simulink model "phase1_PRControl_CIM_Adapt"  (R2024a)
settings: Solver=VariableStepAuto  StartTime=0.0  StopTime=20  FixedStep=1e-6  MaxStep=1e-6  RelTol=1e-6
values from neighbouring files (symbols this model uses):
  alpha_adapt = 100    [phase1_PRControl_CIM_Adapt_init.m]
  Am0_can = sys0_ocf.A    [phase1_PRControl_CIM_Adapt_init.m]
  Bm1_can = sys1_ocf.B    [phase1_PRControl_CIM_Adapt_init.m]
  c_adapt = 0.1    [phase1_PRControl_CIM_Adapt_init.m]
  Cf = 22e-6    (= 2.2e-05)    [phase1_PRControl_CIM_Adapt_init.m]
  Cm0_can = sys0_ocf.C    [phase1_PRControl_CIM_Adapt_init.m]
  E = 1    [phase1_PRControl_CIM_Adapt_init.m]
  freq = 49.5    [phase1_PRControl_CIM_Adapt_init.m]
  L1 = 150e-6    (= 0.00015)    [phase1_PRControl_CIM_Adapt_init.m]
  L2g = L2+Lg    (= 0.00045)    [phase1_PRControl_CIM_Adapt_init.m]
  m_m1 = size(Bm1_can,2)    [phase1_PRControl_CIM_Adapt_init.m]
  n_m0 = size(Am0_can,1)    [phase1_PRControl_CIM_Adapt_init.m]
  p_e = size(E,1)    [phase1_PRControl_CIM_Adapt_init.m]
  PiInit = k0_adapt*eye(m_m1)    [phase1_PRControl_CIM_Adapt_init.m]
  Q_adapt = zeros(m_m1,1)    [phase1_PRControl_CIM_Adapt_init.m]
  R1 = 0.045    [phase1_PRControl_CIM_Adapt_init.m]
  R2g = R2+Rg    (= 0.135)    [phase1_PRControl_CIM_Adapt_init.m]
  Rd = 1    [phase1_PRControl_CIM_Adapt_init.m]
  Theta0 = w0^2    (= 98696.0440109)    [phase1_PRControl_CIM_Adapt_init.m]
  w = 2*pi*freq    (= 311.017672705)    [phase1_PRControl_CIM_Adapt_init.m]
undefined symbols (not defined in the file or in its folder): alfa, Am0, beta, Bm1, C_filter, Cm1, DiscIntNeverNeededParam, Dm1, Down, dt, n0, nu, Th_bar, Up
libraries: fl_lib x34, nesl_utility x23, ee_lib x9, spsSeriesRLCBranchLib x9, cstblocks x7, spsVoltageMeasurementLib x5, spsCurrentMeasurementLib x2, spsDCVoltageSourceLib x2, simulink x2, spsACVoltageSourceLib x1, spsControlledVoltageSourceLib x1, spsBreakerLib x1
(part 1 of 2)
settings Model: Creator=aleks  LastModifiedBy=aleks
settings DataIOCC: ReturnWorkspaceOutputs=off
settings SimscapeCC: SimscapeLogType=all  SimscapeLogOpenViewer=on  SimscapeLogLimitData=off

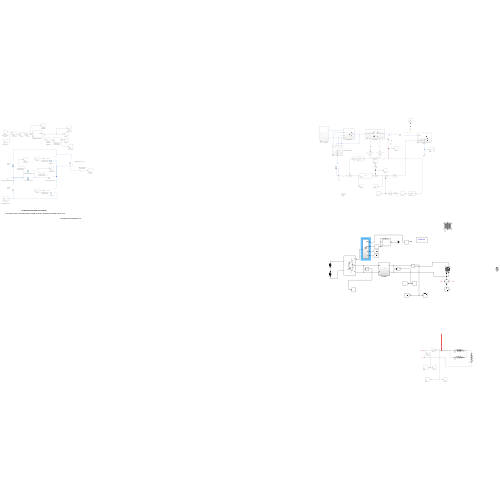
[thumbnail: Simulink's stored preview of the top-level diagram]
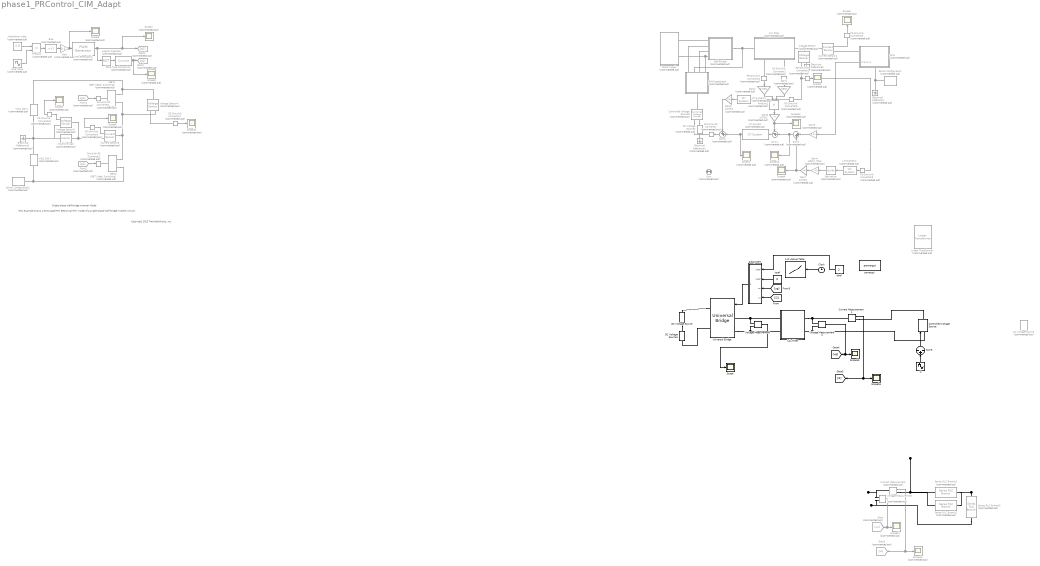
== system phase1_PRControl_CIM_Adapt ==
  note: Single-phase Half-bridge Inverter Model
  note: Copyright 2023 The MathWorks, Inc.
  note: This example shows a Simscape(TM) Electrical(TM) model of a single-phase half-bridge inverter circuit.
  1-D Lookup Table : Lookup_n-D  NumberOfTableDimensions=1  LookupTableObject=''  BreakpointsForDimension1=[0;0.2;0.201;3]  BreakpointsForDimension1FirstPoint=10  BreakpointsForDimension2FirstPoint=10  BreakpointsForDimension1Spacing=12  BreakpointsForDimension2Spacing=12  IndexSearchMethod=Linear search  Table=[0;0;2;2]  DiagnosticForOutOfRangeInput=Error  InternalRulePriority=Speed  RndMeth=Simplest
  AC Voltage Source : spsACVoltageSourceLib/AC Voltage Source  Commented=on  Amplitude=15  Phase=0  Frequency=freq  SampleTime=0  Measurements=None  BusType=swing  Pref=10e3  Qref=0  Qmin=-inf  Qmax=+inf
  Bias : Bias  Commented=on  Bias=1  SaturateOnIntegerOverflow=off
  Clock : Clock
  Controlled Voltage Source2 : fl_lib/Electrical/Electrical Sources/Controlled Voltage Source  Commented=on
  Controlled Voltage Source : spsControlledVoltageSourceLib/Controlled Voltage Source  Initialize=on  Source_Type=AC  Amplitude=0  Phase=0  Frequency=0  Measurements=None
  Current Measurement : spsCurrentMeasurementLib/Current Measurement  Commented=on  PhasorSimulation=off  OutputType=Complex  PSBequivalent=0
  Current Measurement1 : spsCurrentMeasurementLib/Current Measurement  PhasorSimulation=off  OutputType=Complex  PSBequivalent=0
  Current Sensor3 : fl_lib/Electrical/Electrical Sensors/Current Sensor  Commented=on
  Current Sensor4 : fl_lib/Electrical/Electrical Sensors/Current Sensor  Commented=on
  DC Voltage Source : spsDCVoltageSourceLib/DC Voltage Source  Amplitude=20  Measurements=None
  DC Voltage Source1 : spsDCVoltageSourceLib/DC Voltage Source  Amplitude=20  Measurements=None
  DC Voltage Source2 : ee_lib/Additional Components/SPICE Sources/DC Voltage Source  Commented=on  DC=0.3 V
  Data Type Conversion : DataTypeConversion  Commented=on  SaturateOnIntegerOverflow=off  RndMeth=Floor
  Derivative : Derivative  Commented=on
  Electrical Reference{,1..3} (4 alike) : fl_lib/Electrical/Electrical Elements/Electrical Reference  Commented=on
  From1 : From  Commented=on  GotoTag=g1
  From2 : From  Commented=on  GotoTag=g2
  Gain : Gain  Commented=on  Gain=0.5
  Gain1 : Gain  Commented=on  Gain=beta
  Gain2 : Gain  Commented=on  Gain=1-beta
  Gain3 : Gain  Commented=on  Gain=0.01
  Gain4 : Gain  Commented=on  Gain=alfa*C_filter
  Gain5 : Gain  Commented=on  Gain=1/370/2
  Gain6 : Gain  Commented=on  Gain=1/370/2
  Gain7 : Gain  Commented=on  Gain=1/370/2
  Goto : Goto  Commented=on  GotoTag=uo
  Goto1 : Goto  Commented=on  GotoTag=g1
  Goto2 : Goto  Commented=on  GotoTag=g2
  Goto3 : Goto  Commented=on  GotoTag=io
  Grid : Subsystem  Commented=on
      settings: PortSchema="{\"entries\":[{\"content\":{\"sides\":[{\"content\":{\"connectorIds\":[\"LConn1\",\"Out1\"]},\"type\":\"ConnectorPlacement.EquallySpacedRectSide\",\"uuid\":\"60da00de-121a-44fc-8184-3f94833a613b\"},{\"content\":{\"side\":\"RIGHT\"},\"type\":\"ConnectorPlacement.EquallySpacedRectSide\",\"uuid\":\"59ba5a48-7211-453f-9bde-add9e34e0a3d\"},{\"content\":{\"side\":\"TOP\"},\"type\":\"ConnectorPlacement.EquallySpacedRectSide\",\"uuid\":\"7a4f9c1b-94f2-4e83-81a9-ee65f7316222\"},{\"content\":{\"connectorIds\":[\"RConn1\"],\"side\":\"BOTTOM\"},\"type\":\"ConnectorPlacement.EquallySpacedRectSide\",\"uuid\":\"6582cb16-51de-4783-ba21-138861469b9e\"}]},\"type\":\"ConnectorPlacement.EquallySpacedConnector\",\"uuid\":\"6f9c893a-ff6e-44db-92a9-569068b12591\"}],\"packageUris\":[\"http://schema.mathworks.com/mf0/Connector/R2020b\"],\"version\":\"1.0\"}"
  Half-Bridge : Subsystem  Commented=on
  IGBT1 : ee_lib/Semiconductors & Converters/IGBT (Ideal, Switching)  Commented=on  port_option=ee.enum.controlport.ps  Vf=0.8 V  Ron=0.001 Ohm  Goff=1e-5 1/Ohm  Vth=0.5 V  diode_param=2  diode_Vf=0.8 V  diode_Ron=0.001 Ohm  diode_Goff=1e-5 1/Ohm  diode_C=50e-9 F  diode_iRM=-235 A  diode_iF=300 A  diode_idot=-50 A/us  diode_trr_param=1  diode_trr_factor=3  diode_trr=15 us  diode_Qrr=1500 s*uA  ice_specify=off  ice_priority=None  ice=0 A  ice_nominal_specify=off  ice_nominal_value=1  ice_nominal_unit=A  vce_specify=off  vce_priority=None  vce=0 V  vce_nominal_specify=off  vce_nominal_value=1  vce_nominal_unit=V  vge_specify=off  vge_priority=None  vge=0 V  vge_nominal_specify=off  vge_nominal_value=1  vge_nominal_unit=V  thermal_loss_option=ee.enum.converters.thermalLossOption.constantvalues  Von_data=[0, .1, .6, .8, 1, 1.3, 1.6, 2, 2.4; 0, .1, .7, 1, 1.2, 1.5, 1.9, 2.4, 2.8] V  Tj=[298.15, 398.15] K  Iout_data=[0, .1, 1, 5, 10, 20, 40, 70, 100] A  Eon_data=[0, .0024, .024, .12, .2, .48, 1.04, 2.16, 3.24; 0, .003, .03, .15, .25, .6, 1.3, 2.7, 4.05] * 1e-3 J  Eoff_data=[0, .0007, .0066, .033, .066, .17, .33, .83, 1.5; 0, .001, .01, .05, .1, .25, .5, 1.2, 2.2] * 1e-3 J  Eon_data_3D=[zeros(2, 9, 3)] J  Eoff_data_3D=[zeros(2, 9, 3)] J  Tj_loss=[298.15, 398.15] K  Iout_data_loss=[0, .1, 1, 5, 10, 20, 40, 70, 100] A  tabulateWithVce=false  Vce_loss=[0, 150, 300] V  Eon_scalar=22.86e-3 J  Eoff_scalar=17.14e-3 J  Voff=300 V  Iout_scalar=600 A  useCurrentFromPreviousCycle=false  useVoltageFromPreviousCycle=false  diodeModelType=ee.enum.converters.diodeModelType.pwl  diodeTableType=ee.enum.diode.tableType.IfMat  diode_ReverseIVType=ee.enum.diode.diodeReverseIV.constant  diode_IfMat=[.07, .12, .19, 1.75, 4.24, 7.32, 11.2; .16, .3, .72, 2.14, 4.02, 6.35, 9.12] A  diode_VfMat=[.9, 1.15, 1.25, 1.5, 1.75, 2.17, 2.6, 2.85; .58, .68, .75, 1.1, 1.38, 1.77, 2.27, 2.7] V  diode_TjVec=[25, 125] degC  diode_VfVec=[.5, .7, .9, 1.3, 1.7, 2.1, 2.5] V  diode_IfVec=[.1, .2, .5, 1, 2, 4, 7, 10] A  diode_IrMat=[1e-06, 2e-06, 5e-06, 1e-05, 2.5e-05, 5e-05, .0001; 2e-06, 5e-06, 1e-05, 4e-05, 8e-05, .0002, .0005] A  diode_VrMat=[10, 100, 200, 250, 300, 325, 350; 10, 70, 160, 220, 270, 300, 320] V  diode_VrVec=[10, 20, 40, 50, 70, 80, 100] V  diode_IrVec=[1e-06, 2e-06, 5e-06, 1e-05, 2e-05, 5e-05, .0001] A  diode_Vr=-600 V  diode_Ls=150 nH  diode_Erec=0.03 J  diode_rec_loss_model=ee.enum.diode.reverseRecoveryModel.fixed  diode_ErecVal=0 J  diode_scaleWithIandV=true  diode_ErecMat=zeros(2, 3) J  diode_TjrecVec=[298.15, 398.15] K  diode_IfrecVec=[.1, 1, 10] A  diode_IrecVal=10 A  diode_VrecVal=10 V  diode_tFilter=1 / 1000 / 100 s  thermal_network_parameterization=ee.enum.thermalNetworkTopology.external  Rth=[.08, .5] K/W  Rth_Cauer=[.08, .1, .5] K/W  Rth_Foster=[.08, .14, .22, .16] K/W  thermal_mass_parameterization=ee.enum.thermalNetwork.timeconstant  thermal_mass=[.01, .5] J/K  thermal_mass_Cauer=[.01, .1, .5] J/K  thermal_mass_Foster=[.001, .005, .05, .5] J/K  thermal_time_constant=[.001, .2] s  thermal_time_constant_Cauer=[.001, .1, .2] s  thermal_time_constant_Foster=[7e-05, .0007, .01, .08] s  thermal_mass_initial_temperatures=[25, 25] degC  thermal_mass_initial_temperatures_Cauer=[25, 25, 25] degC  junction_thermal_mass=0.01 J/K  Tvec_initial_Foster=[25, 25, 25, 25] degC  no_thermal_network=0  junction_temperature_specify=off  junction_temperature_priority=None  junction_temperature=25 degC  junction_temperature_nominal_specify=off  junction_temperature_nominal_value=1  junction_temperature_nominal_unit=degC  Qj_specify=off  Qj_priority=None  Qj=0 W  Qj_nominal_specify=off  Qj_nominal_value=1  Qj_nominal_unit=W  accumulatedSwitchingLosses_specify=off  accumulatedSwitchingLosses_priority=None  accumulatedSwitchingLosses=0 J
  IGBT2 : ee_lib/Semiconductors & Converters/IGBT (Ideal, Switching)  Commented=on  port_option=ee.enum.controlport.ps  Vf=0.8 V  Ron=0.001 Ohm  Goff=1e-5 1/Ohm  Vth=0.5 V  diode_param=2  diode_Vf=0.8 V  diode_Ron=0.001 Ohm  diode_Goff=1e-5 1/Ohm  diode_C=50e-9 F  diode_iRM=-235 A  diode_iF=300 A  diode_idot=-50 A/us  diode_trr_param=1  diode_trr_factor=3  diode_trr=15 us  diode_Qrr=1500 s*uA  ice_specify=off  ice_priority=None  ice=0 A  ice_nominal_specify=off  ice_nominal_value=1  ice_nominal_unit=A  vce_specify=off  vce_priority=None  vce=0 V  vce_nominal_specify=off  vce_nominal_value=1  vce_nominal_unit=V  vge_specify=off  vge_priority=None  vge=0 V  vge_nominal_specify=off  vge_nominal_value=1  vge_nominal_unit=V  thermal_loss_option=ee.enum.converters.thermalLossOption.constantvalues  Von_data=[0, .1, .6, .8, 1, 1.3, 1.6, 2, 2.4; 0, .1, .7, 1, 1.2, 1.5, 1.9, 2.4, 2.8] V  Tj=[298.15, 398.15] K  Iout_data=[0, .1, 1, 5, 10, 20, 40, 70, 100] A  Eon_data=[0, .0024, .024, .12, .2, .48, 1.04, 2.16, 3.24; 0, .003, .03, .15, .25, .6, 1.3, 2.7, 4.05] * 1e-3 J  Eoff_data=[0, .0007, .0066, .033, .066, .17, .33, .83, 1.5; 0, .001, .01, .05, .1, .25, .5, 1.2, 2.2] * 1e-3 J  Eon_data_3D=[zeros(2, 9, 3)] J  Eoff_data_3D=[zeros(2, 9, 3)] J  Tj_loss=[298.15, 398.15] K  Iout_data_loss=[0, .1, 1, 5, 10, 20, 40, 70, 100] A  tabulateWithVce=false  Vce_loss=[0, 150, 300] V  Eon_scalar=22.86e-3 J  Eoff_scalar=17.14e-3 J  Voff=300 V  Iout_scalar=600 A  useCurrentFromPreviousCycle=false  useVoltageFromPreviousCycle=false  diodeModelType=ee.enum.converters.diodeModelType.pwl  diodeTableType=ee.enum.diode.tableType.IfMat  diode_ReverseIVType=ee.enum.diode.diodeReverseIV.constant  diode_IfMat=[.07, .12, .19, 1.75, 4.24, 7.32, 11.2; .16, .3, .72, 2.14, 4.02, 6.35, 9.12] A  diode_VfMat=[.9, 1.15, 1.25, 1.5, 1.75, 2.17, 2.6, 2.85; .58, .68, .75, 1.1, 1.38, 1.77, 2.27, 2.7] V  diode_TjVec=[25, 125] degC  diode_VfVec=[.5, .7, .9, 1.3, 1.7, 2.1, 2.5] V  diode_IfVec=[.1, .2, .5, 1, 2, 4, 7, 10] A  diode_IrMat=[1e-06, 2e-06, 5e-06, 1e-05, 2.5e-05, 5e-05, .0001; 2e-06, 5e-06, 1e-05, 4e-05, 8e-05, .0002, .0005] A  diode_VrMat=[10, 100, 200, 250, 300, 325, 350; 10, 70, 160, 220, 270, 300, 320] V  diode_VrVec=[10, 20, 40, 50, 70, 80, 100] V  diode_IrVec=[1e-06, 2e-06, 5e-06, 1e-05, 2e-05, 5e-05, .0001] A  diode_Vr=-600 V  diode_Ls=150 nH  diode_Erec=0.03 J  diode_rec_loss_model=ee.enum.diode.reverseRecoveryModel.fixed  diode_ErecVal=0 J  diode_scaleWithIandV=true  diode_ErecMat=zeros(2, 3) J  diode_TjrecVec=[298.15, 398.15] K  diode_IfrecVec=[.1, 1, 10] A  diode_IrecVal=10 A  diode_VrecVal=10 V  diode_tFilter=1 / 1000 / 100 s  thermal_network_parameterization=ee.enum.thermalNetworkTopology.external  Rth=[.08, .5] K/W  Rth_Cauer=[.08, .1, .5] K/W  Rth_Foster=[.08, .14, .22, .16] K/W  thermal_mass_parameterization=ee.enum.thermalNetwork.timeconstant  thermal_mass=[.01, .5] J/K  thermal_mass_Cauer=[.01, .1, .5] J/K  thermal_mass_Foster=[.001, .005, .05, .5] J/K  thermal_time_constant=[.001, .2] s  thermal_time_constant_Cauer=[.001, .1, .2] s  thermal_time_constant_Foster=[7e-05, .0007, .01, .08] s  thermal_mass_initial_temperatures=[25, 25] degC  thermal_mass_initial_temperatures_Cauer=[25, 25, 25] degC  junction_thermal_mass=0.01 J/K  Tvec_initial_Foster=[25, 25, 25, 25] degC  no_thermal_network=0  junction_temperature_specify=off  junction_temperature_priority=None  junction_temperature=25 degC  junction_temperature_nominal_specify=off  junction_temperature_nominal_value=1  junction_temperature_nominal_unit=degC  Qj_specify=off  Qj_priority=None  Qj=0 W  Qj_nominal_specify=off  Qj_nominal_value=1  Qj_nominal_unit=W  accumulatedSwitchingLosses_specify=off  accumulatedSwitchingLosses_priority=None  accumulatedSwitchingLosses=0 J
  Idref : Constant  Value=2
  Inductive load : fl_lib/Electrical/Electrical Elements/Inductor  Commented=on  l=0.005 H  r=1 Ohm  g=0 1/Ohm  i_specify=off  i_priority=None  i=0 A  i_nominal_specify=off  i_nominal_value=1  i_nominal_unit=A  v_specify=off  v_priority=None  v=0 V  v_nominal_specify=off  v_nominal_value=1  v_nominal_unit=V  i_L_specify=off  i_L_priority=High  i_L=0 A  i_L_nominal_specify=off  i_L_nominal_value=1  i_L_nominal_unit=A
  Iqref : Constant  Value=0
  LCL Filter : Subsystem
  LCL filter : Subsystem  Commented=on
      settings: PortSchema="{\"entries\":[{\"content\":{\"sides\":[{\"content\":{\"connectorIds\":[\"LConn1\"]},\"type\":\"ConnectorPlacement.EquallySpacedRectSide\",\"uuid\":\"8b3831d8-2af2-4e09-98b8-6e5c23c190ef\"},{\"content\":{\"connectorIds\":[\"RConn1\"],\"side\":\"RIGHT\"},\"type\":\"ConnectorPlacement.EquallySpacedRectSide\",\"uuid\":\"7bed20d9-2cda-4fdb-ba4d-dd3d87999dd3\"},{\"content\":{\"side\":\"TOP\"},\"type\":\"ConnectorPlacement.EquallySpacedRectSide\",\"uuid\":\"ddfcc6a1-9f78-4bcc-aaa8-1a77e264e72f\"},{\"content\":{\"connectorIds\":[\"RConn2\",\"RConn3\"],\"side\":\"BOTTOM\"},\"type\":\"ConnectorPlacement.EquallySpacedRectSide\",\"uuid\":\"a456a5b4-e9ed-42f1-ab5a-c7df7a648cd2\"}]},\"type\":\"ConnectorPlacement.EquallySpacedConnector\",\"uuid\":\"6c992da4-40d5-4809-a728-0540f255a39b\"}],\"packageUris\":[\"http://schema.mathworks.com/mf0/Connector/R2020b\"],\"version\":\"1.0\"}"
  LTI System : cstblocks/LTI System  Commented=on  sys=Gpr  IC=[]  PadeOrder=0
  LTI System1 : cstblocks/LTI System  Commented=on  sys=Gfffilter  IC=[]  PadeOrder=0
  LTI System2 : cstblocks/LTI System  Commented=on  sys=Gfffilter  IC=[]  PadeOrder=0
  Linear Transformer : spsLinearTransformerLib/Linear Transformer  Commented=on  UNITS=pu  NominalPower=[ 45 50 ]  winding1="[ 15/sqrt(2)  0.002  0.01 ]"  winding2="[ 230  0.002  0.01 ]"  ThreeWindings=off  winding3=[ 315e3 0.002 0.08 ]  RmLm=[ 500 500 ]  Measurements=None  DataType=off
  Logical Operator : Logic  Commented=on  Operator=NOT  AllPortsSameDT=off  OutDataTypeStr=boolean
  Modulation Index : Constant  Commented=on  Value=0.8
  PS-Simulink Converter{1..9} (9 alike) : nesl_utility/PS-Simulink Converter  Commented=on  PhysicalDomain=network_engine_domain  SubClassName=ps_output  LeftPortType=input  RightPortType=output  PseudoPeriodic=off  Frequencies=[]  VectorFormat=inherit  Unit=inherit  AffineConversion=off
  PWM Generator1 : eePwmGenerator/PWM Generator  Commented=on  CarrCount=Up-Down  Tper=1/2/2000  Tdelay=0  Ts=0
  PWM generator : Subsystem  Commented=on
  Power supply : Subsystem  Commented=on
  Product : Product  Commented=on  RndMeth=Zero
  Product1 : Product  Commented=on
  Scope : Scope
  Scope{1..14} (14 alike) : Scope  Commented=on
  Scope15 : Scope
  Scope16 : Scope
  Series RLC Branch1 : spsSeriesRLCBranchLib/Series RLC Branch  Commented=on  LConnTagsString=__new0  RConnTagsString=__new0  BranchType=L  Resistance=0.053  Inductance=5e-3  SetiL0=off  InitialCurrent=0  Capacitance=1e-6  Setx0=off  InitialVoltage=0  Measurements=None
  Series RLC Branch2 : spsSeriesRLCBranchLib/Series RLC Branch  Commented=on  LConnTagsString=__new0  RConnTagsString=__new0  BranchType=R  Resistance=500  Inductance=500e-6  SetiL0=off  InitialCurrent=0  Capacitance=1e-6  Setx0=off  InitialVoltage=0  Measurements=None
  Series RLC Branch3 : spsSeriesRLCBranchLib/Series RLC Branch  Commented=on  LConnTagsString=__new0  RConnTagsString=__new0  BranchType=R  Resistance=5  Inductance=500e-6  SetiL0=off  InitialCurrent=0  Capacitance=1e-6  Setx0=off  InitialVoltage=0  Measurements=None
  Simulink-PS Converter : nesl_utility/Simulink-PS Converter  Commented=on  PhysicalDomain=network_engine_domain  SubClassName=ps_input  LeftPortType=input  RightPortType=output  PseudoPeriodic=off  Frequencies=[]  NoiseDistribution=none  NoiseParameters=[]  Unit=1  AffineConversion=off  FilteringAndDerivatives=provide  SimscapeFilterOrder=1  InputFilterTimeConstant=0.001  UdotUserProvided=0
  Simulink-PS Converter1 : nesl_utility/Simulink-PS Converter  Commented=on  PhysicalDomain=network_engine_domain  SubClassName=ps_input  LeftPortType=input  RightPortType=output  PseudoPeriodic=off  Frequencies=[]  NoiseDistribution=none  NoiseParameters=[]  Unit=1  AffineConversion=off  FilteringAndDerivatives=provide  SimscapeFilterOrder=1  InputFilterTimeConstant=0.001  UdotUserProvided=0
  Simulink-PS Converter2 : nesl_utility/Simulink-PS Converter  Commented=on  PhysicalDomain=network_engine_domain  SubClassName=ps_input  LeftPortType=input  RightPortType=output  PseudoPeriodic=off  Frequencies=[]  NoiseDistribution=none  NoiseParameters=[]  Unit=1  AffineConversion=off  FilteringAndDerivatives=provide  SimscapeFilterOrder=1  InputFilterTimeConstant=0.001  UdotUserProvided=0
  Sine Wave : Sin  Commented=on  Frequency=2*pi*50  SampleTime=0
  Solver Configuration : nesl_utility/Solver Configuration  Commented=on  PhysicalDomain=network_engine_domain  SubClassName=solver  LeftPortType=input  RightPortType=generic  Tones=[]  Harmonics=[]  SimulateNoise=off  Profile=off  UseLocalSampling=off  EnableSwitchedLinearOptims=on  FrequencyDomain=off  UseCCode=off  RelTol=0.001  AbsTol=0.001  MinStep=1e-09  ToWorkspace=off  RevertToSquareIcSolve=off  NumHomotopyIterations=100  PhasorMode=off  PhasorModeNumHarmonics=1  ConsistencySolver=NEWTON_XTOL_AFTER_FTOL  IndexReductionMethod=DerivativeReplacement  DoDC=off  ResidualTolerance=1e-09  ConsistencyTolSource=GLOBAL  ConsistencyAbsTol=0.001  ConsistencyRelTol=0.001  ConsistencyTolFactor=0.001  UseLocalSolver=off  LocalSolverChoice=NE_BACKWARD_EULER_ADVANCER  ResolveIndetEquations=on  FunctionEvalNumThread=1  LocalSolverSampleTime=0.001  DoFixedCost=off  MaxNonlinIter=3  MaxModeIter=2  ComputeImpulses=off  ImpulseIterations=2  LinearAlgebra=auto  LinearAlgebraNumThread=0  EquationFormulation=NE_TIME_EF  DelaysMemoryBudget=1024  AutomaticFiltering=on  FilteringTimeConstant=0.001  PartitionStorageMethod=AS_NEEDED  PartitionMemoryBudget=1024  PartitionMethod=ROBUST  MultibodyUseLocalSolver=off  MultibodyLocalSolverChoice=ODE1  MultibodyLocalSolverSampleTime=0.001
  Solver Configuration2 : nesl_utility/Solver Configuration  Commented=on  PhysicalDomain=network_engine_domain  SubClassName=solver  LeftPortType=input  RightPortType=generic  Tones=[]  Harmonics=[]  SimulateNoise=off  Profile=off  UseLocalSampling=off  EnableSwitchedLinearOptims=on  FrequencyDomain=off  UseCCode=off  RelTol=0.001  AbsTol=1e-06  MinStep=1e-09  ToWorkspace=off  RevertToSquareIcSolve=off  NumHomotopyIterations=100  PhasorMode=off  PhasorModeNumHarmonics=1  ConsistencySolver=NEWTON_FTOL  IndexReductionMethod=DerivativeReplacement  DoDC=off  ResidualTolerance=1e-09  ConsistencyTolSource=GLOBAL  ConsistencyAbsTol=0.001  ConsistencyRelTol=0.001  ConsistencyTolFactor=0.001  UseLocalSolver=off  LocalSolverChoice=NE_BACKWARD_EULER_ADVANCER  ResolveIndetEquations=on  FunctionEvalNumThread=1  LocalSolverSampleTime=5e-05  DoFixedCost=off  MaxNonlinIter=3  MaxModeIter=2  ComputeImpulses=off  ImpulseIterations=1  LinearAlgebra=Sparse  LinearAlgebraNumThread=0  EquationFormulation=NE_TIME_EF  DelaysMemoryBudget=1024  AutomaticFiltering=on  FilteringTimeConstant=0.001  PartitionStorageMethod=AS_NEEDED  PartitionMemoryBudget=1024  PartitionMethod=FAST  MultibodyUseLocalSolver=off  MultibodyLocalSolverChoice=ODE1  MultibodyLocalSolverSampleTime=0.001
  Subsystem : Subsystem
  Sum : Sum  Commented=on  Inputs=+|+
  Sum1 : Sum  Commented=on  Inputs=-+|
  Sum2 : Sum  Commented=on  Inputs=|++
  Sum3 : Sum  Commented=on  Inputs=++|
  Sum5 : Sum  Inputs=-|+|-
  Universal Bridge : spsUniversalBridgeLib/Universal Bridge  Arms=2  SnubberResistance=1e5  SnubberCapacitance=inf  Device=IGBT / Diodes  Ron=1e-3  Lon=0  ForwardVoltages="[  0  0  ]"  ForwardVoltage=0  GTOparameters=[ 10e-6 , 20e-6 ]  IGBTparameters=[ 1e-6 , 2e-6 ]  Measurements=None  Measurements_2=None  converterType=Rectifier
  Vdc1 100 V : fl_lib/Electrical/Electrical Sources/DC Voltage Source  Commented=on  v0=100 V
  Vdc2 100 V : fl_lib/Electrical/Electrical Sources/DC Voltage Source  Commented=on  v0=100 V
  Voltage Measurement : spsVoltageMeasurementLib/Voltage Measurement  PhasorSimulation=off  OutputType=Complex  PSBequivalent=0
  Voltage Measurement1 : spsVoltageMeasurementLib/Voltage Measurement  Commented=on  PhasorSimulation=off  OutputType=Complex  PSBequivalent=0
  Voltage Measurement2 : spsVoltageMeasurementLib/Voltage Measurement  PhasorSimulation=off  OutputType=Complex  PSBequivalent=0
  Voltage Sensor : fl_lib/Electrical/Electrical Sensors/Voltage Sensor  Commented=on
  Voltage Sensor3 : fl_lib/Electrical/Electrical Sensors/Voltage Sensor  Commented=on
  Voltage Sensor4 : fl_lib/Electrical/Electrical Sensors/Voltage Sensor  Commented=on
  powergui : spspowerguiLib/powergui  Priority=1  SimulationMode=Continuous  SampleTime=10e-6  frequency=60  Iterations=50  frequencyindice=0  Pbase=100e6  ErrMax=1e-4  UnitsV=kV  UnitsW=MW  buscounter=0  FunctionMessages=off  echomessages=off  EnableUseOfTLC=off  CurrentSourceSwitches=off  DisableSnubberDevices=off  DisableRonSwitches=off  DisableVfSwitches=off  DisplayEquations=off  AutomaticDiscreteSolvers=off  SolverType=Tustin/Backward Euler (TBE)  Interpol=off  ExternalGateDelay=off  methode=off  Ts=100  x0status=blocks  SPID=on  SwTol=0  HookPort=off  NonlinearTolerance=1e-4  nMaxIteration=100  ContinueOnMaxIteration=off  RestoreLinks=warning  ResistiveCurrentMeasurement=off  Frange=[0:2:500]  Ylog=off  Xlog=on  ShowGrid=off  save=off  variable=ZData  structure=0  ZoomFFT=off  StartTime=0.0  cycles=1  DisplayStyle=1  fundamental=60  FreqAxis=off  MaxFrequency=1000  frequencyindicesteady=1  RmsSteady=1  display=off
  w : Sin  Amplitude=15  Frequency=w  SampleTime=0
  wires:
  PS-Simulink Converter2/1 -> Scope2/1
  Bias/1 -> Gain/1
  Product/1 -> Bias/1
  From1/1 -> Simulink-PS Converter1/1
  Logical Operator/1 -> Data Type Conversion/1
  Sine Wave/1 -> Product/2
  PS-Simulink Converter5/1 -> Scope6/1
  From2/1 -> Simulink-PS Converter2/1
  PS-Simulink Converter6/1 -> Scope5/1
  Modulation Index/1 -> Product/1
  Data Type Conversion/1 -> Scope9/1, Goto2/1
  PWM Generator1/1 -> Scope7/1, Goto1/1, Logical Operator/1
  Gain/1 -> Scope8/1, PWM Generator1/1
  PS-Simulink Converter7/1 -> Scope10/1
  PS-Simulink Converter3/1 -> Scope3/1
  PS-Simulink Converter1/1 -> Gain1/1
  PS-Simulink Converter4/1 -> Gain2/1
  Gain2/1 -> Product1/1
  Gain1/1 -> Product1/2
  Grid/1(sinewave) -> Gain3/1
  Gain3/1 -> Sum2/1
  Gain6/1 -> Sum1/1, Scope13/1
  Sum1/1 -> LTI System/1
  Derivative/1 -> Gain4/1
  Gain7/1 -> Sum2/2, Scope4/1
  Sum2/1 -> Scope12/1, Sum1/2
  LTI System/1 -> Sum3/2, Scope1/1
  PS-Simulink Converter8/1 -> LTI System1/1
  Sum3/1 -> Simulink-PS Converter/1
  Gain5/1 -> Sum3/1
  Product1/1 -> Gain6/1
  LTI System1/1 -> Gain5/1
  PS-Simulink Converter9/1 -> LTI System2/1
  LTI System2/1 -> Derivative/1
  Gain4/1 -> Gain7/1
  Voltage Measurement/1 -> Scope/1
  Subsystem/1(1) -> Universal Bridge/1
  [i2] -> Subsystem/4(io)
  [ug] -> Subsystem/3(uo)
  Current Measurement/1 -> Scope14/1, Goto3/1
  Voltage Measurement1/1 -> Goto/1, Scope11/1
  Voltage Measurement2/1 -> [ug], Scope15/1
  Current Measurement1/1 -> Scope16/1, [i2]
  w/1 -> Sum5/2
  ? -> ?
  ? -> ?
  Sum5/1 -> Controlled Voltage Source/1
  Iqref/1 -> Subsystem/2(iqref)
  Idref/1 -> Subsystem/1(idref)
  Clock/1 -> 1-D Lookup Table/1
  connections:
  Voltage Sensor/LConn1 -- Current Sensor4/LConn1 -- LCL filter/RConn1
  Voltage Sensor/RConn1 -- PS-Simulink Converter9/LConn1 -- PS-Simulink Converter8/LConn1 -- PS-Simulink Converter2/LConn1
  Solver Configuration2/RConn1 -- Vdc2 100 V/RConn1 -- IGBT2/RConn2
  Vdc1 100 V/RConn1 -- Vdc2 100 V/LConn1 -- Electrical Reference2/LConn1 -- Inductive load/RConn1 -- Voltage Sensor3/RConn2
  Current Sensor3/RConn2 -- Inductive load/LConn1 -- Voltage Sensor3/LConn1
  IGBT2/RConn1 -- Current Sensor3/LConn1 -- IGBT1/RConn2 -- Voltage Sensor4/RConn2
  IGBT1/RConn1 -- Voltage Sensor4/LConn1 -- Vdc1 100 V/LConn1
  PS-Simulink Converter5/LConn1 -- Current Sensor3/RConn1
  PS-Simulink Converter6/LConn1 -- Voltage Sensor3/RConn1
  IGBT2/LConn1 -- Simulink-PS Converter2/RConn1
  IGBT1/LConn1 -- Simulink-PS Converter1/RConn1
  Voltage Sensor4/RConn1 -- PS-Simulink Converter7/LConn1
  Controlled Voltage Source2/LConn1 -- PWM generator/LConn1
  Half-Bridge/RConn1 -- PWM generator/RConn2 -- LCL filter/LConn1
  Half-Bridge/LConn2 -- PWM generator/RConn1
  PWM generator/RConn3 -- Half-Bridge/LConn3
  Voltage Sensor/RConn2 -- Electrical Reference3/LConn1
  PS-Simulink Converter3/LConn1 -- Current Sensor4/RConn1
  Current Sensor4/RConn2 -- Grid/LConn1
  Electrical Reference/LConn1 -- Solver Configuration/RConn1 -- Grid/RConn1
  PWM generator/RConn4 -- Power supply/RConn2 -- Half-Bridge/LConn4
  Half-Bridge/LConn1 -- Power supply/RConn1
  DC Voltage Source2/RConn1 -- Electrical Reference1/LConn1
  Controlled Voltage Source2/RConn2 -- DC Voltage Source2/LConn1
  PS-Simulink Converter4/LConn1 -- LCL filter/RConn2
  LCL filter/RConn3 -- PS-Simulink Converter1/LConn1
  Controlled Voltage Source2/RConn1 -- Simulink-PS Converter/RConn1
  Universal Bridge/RConn1 -- DC Voltage Source/RConn1
  Universal Bridge/RConn2 -- DC Voltage Source1/LConn1
  Voltage Measurement/LConn1 -- LCL Filter/LConn1 -- Universal Bridge/LConn1
  Voltage Measurement2/LConn2 -- Controlled Voltage Source/LConn1 -- LCL Filter/RConn2
  DC Voltage Source/LConn1 -- DC Voltage Source1/RConn1
  Voltage Measurement1/LConn1 -- Current Measurement/LConn1
  Series RLC Branch1/LConn1 -- Series RLC Branch2/LConn1 -- Current Measurement/RConn1
  Series RLC Branch3/LConn1 -- Series RLC Branch1/RConn1 -- Series RLC Branch2/RConn1
  Series RLC Branch3/RConn1 -- Voltage Measurement1/LConn2
  Voltage Measurement2/LConn1 -- LCL Filter/RConn1 -- Current Measurement1/LConn1
  Voltage Measurement/LConn2 -- LCL Filter/LConn2 -- Universal Bridge/LConn2
  Current Measurement1/RConn1 -- Controlled Voltage Source/RConn1

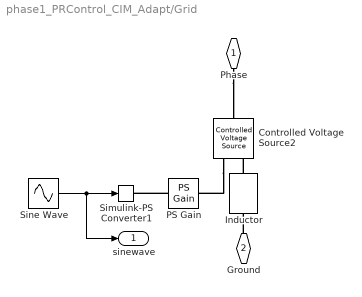
== system phase1_PRControl_CIM_Adapt/Grid ==
  Controlled Voltage Source2 : fl_lib/Electrical/Electrical Sources/Controlled Voltage Source
  Inductor : fl_lib/Electrical/Electrical Elements/Inductor  l=5e-3 H  r=0.35 Ohm  g=1e-9 1/Ohm  i_specify=off  i_priority=None  i=0 A  i_nominal_specify=off  i_nominal_value=1  i_nominal_unit=A  v_specify=off  v_priority=None  v=0 V  v_nominal_specify=off  v_nominal_value=1  v_nominal_unit=V  i_L_specify=off  i_L_priority=High  i_L=0 A  i_L_nominal_specify=off  i_L_nominal_value=1  i_L_nominal_unit=A
  PS Gain : fl_lib/Physical Signals/Functions/PS Gain  gain=220
  Simulink-PS Converter1 : nesl_utility/Simulink-PS Converter  PhysicalDomain=network_engine_domain  SubClassName=ps_input  LeftPortType=input  RightPortType=output  PseudoPeriodic=off  Frequencies=[]  NoiseDistribution=none  NoiseParameters=[]  Unit=1  AffineConversion=off  FilteringAndDerivatives=filter  SimscapeFilterOrder=1  InputFilterTimeConstant=0.0001  UdotUserProvided=0
  Sine Wave : Sin  Frequency=2*pi*50  SampleTime=0
  Phase : PMIOPort  Side=Left
  Ground : PMIOPort  Port=2  Side=Right
  sinewave : Outport
  wires:
  Sine Wave/1 -> sinewave/1, Simulink-PS Converter1/1
  connections:
  Phase/RConn1 -- Controlled Voltage Source2/LConn1
  Controlled Voltage Source2/RConn1 -- PS Gain/RConn1
  Inductor/LConn1 -- Controlled Voltage Source2/RConn2
  Ground/RConn1 -- Inductor/RConn1
  PS Gain/LConn1 -- Simulink-PS Converter1/RConn1

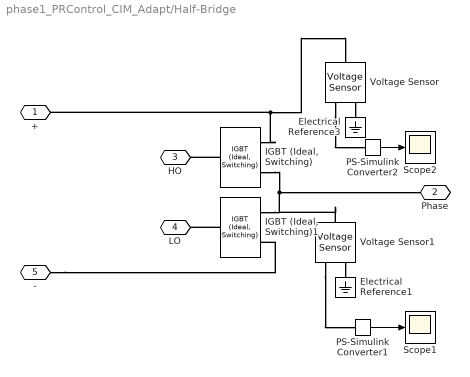
== system phase1_PRControl_CIM_Adapt/Half-Bridge ==
  Electrical Reference1 : fl_lib/Electrical/Electrical Elements/Electrical Reference
  Electrical Reference3 : fl_lib/Electrical/Electrical Elements/Electrical Reference
  "IGBT (Ideal, Switching)" : ee_lib/Semiconductors & Converters/IGBT (Ideal, Switching)  port_option=ee.enum.controlport.elec  Vf=0.8 V  Ron=0.001 Ohm  Goff=1e-5 1/Ohm  Vth=0.5 V  diode_param=ee.enum.semiconductors.protectionDiode.nodynamics  diode_Vf=0.8 V  diode_Ron=0.001 Ohm  diode_Goff=1e-5 1/Ohm  diode_C=50e-9 F  diode_iRM=-235 A  diode_iF=300 A  diode_idot=-50 A/us  diode_trr_param=ee.enum.converters.diodeReverseParam.trr_factor  diode_trr_factor=3  diode_trr=15 us  diode_Qrr=1500 s*uA  ice_specify=off  ice_priority=None  ice=0 A  ice_nominal_specify=off  ice_nominal_value=1  ice_nominal_unit=A  vce_specify=off  vce_priority=None  vce=0 V  vce_nominal_specify=off  vce_nominal_value=1  vce_nominal_unit=V  vge_specify=off  vge_priority=None  vge=0 V  vge_nominal_specify=off  vge_nominal_value=1  vge_nominal_unit=V  thermal_loss_option=ee.enum.converters.thermalLossOption.constantvalues  Von_data=[0, .1, .6, .8, 1, 1.3, 1.6, 2, 2.4; 0, .1, .7, 1, 1.2, 1.5, 1.9, 2.4, 2.8] V  Tj=[298.15, 398.15] K  Iout_data=[0, .1, 1, 5, 10, 20, 40, 70, 100] A  Eon_data=[0, .0024, .024, .12, .2, .48, 1.04, 2.16, 3.24; 0, .003, .03, .15, .25, .6, 1.3, 2.7, 4.05] * 1e-3 J  Eoff_data=[0, .0007, .0066, .033, .066, .17, .33, .83, 1.5; 0, .001, .01, .05, .1, .25, .5, 1.2, 2.2] * 1e-3 J  Eon_data_3D=[zeros(2, 9, 3)] J  Eoff_data_3D=[zeros(2, 9, 3)] J  Tj_loss=[298.15, 398.15] K  Iout_data_loss=[0, .1, 1, 5, 10, 20, 40, 70, 100] A  tabulateWithVce=false  Vce_loss=[0, 150, 300] V  Eon_scalar=22.86e-3 J  Eoff_scalar=17.14e-3 J  Voff=300 V  Iout_scalar=600 A  useCurrentFromPreviousCycle=false  useVoltageFromPreviousCycle=false  diodeModelType=ee.enum.converters.diodeModelType.pwl  diodeTableType=ee.enum.diode.tableType.IfMat  diode_ReverseIVType=ee.enum.diode.diodeReverseIV.constant  diode_IfMat=[.07, .12, .19, 1.75, 4.24, 7.32, 11.2; .16, .3, .72, 2.14, 4.02, 6.35, 9.12] A  diode_VfMat=[.9, 1.15, 1.25, 1.5, 1.75, 2.17, 2.6, 2.85; .58, .68, .75, 1.1, 1.38, 1.77, 2.27, 2.7] V  diode_TjVec=[25, 125] degC  diode_VfVec=[.5, .7, .9, 1.3, 1.7, 2.1, 2.5] V  diode_IfVec=[.1, .2, .5, 1, 2, 4, 7, 10] A  diode_IrMat=[1e-06, 2e-06, 5e-06, 1e-05, 2.5e-05, 5e-05, .0001; 2e-06, 5e-06, 1e-05, 4e-05, 8e-05, .0002, .0005] A  diode_VrMat=[10, 100, 200, 250, 300, 325, 350; 10, 70, 160, 220, 270, 300, 320] V  diode_VrVec=[10, 20, 40, 50, 70, 80, 100] V  diode_IrVec=[1e-06, 2e-06, 5e-06, 1e-05, 2e-05, 5e-05, .0001] A  diode_Vr=-600 V  diode_Ls=150 nH  diode_Erec=0.03 J  diode_rec_loss_model=ee.enum.diode.reverseRecoveryModel.fixed  diode_ErecVal=0 J  diode_scaleWithIandV=true  diode_ErecMat=zeros(2, 3) J  diode_TjrecVec=[298.15, 398.15] K  diode_IfrecVec=[.1, 1, 10] A  diode_IrecVal=10 A  diode_VrecVal=10 V  diode_tFilter=1 / 1000 / 100 s  thermal_network_parameterization=ee.enum.thermalNetworkTopology.external  Rth=[.08, .5] K/W  Rth_Cauer=[.08, .1, .5] K/W  Rth_Foster=[.08, .14, .22, .16] K/W  thermal_mass_parameterization=ee.enum.thermalNetwork.timeconstant  thermal_mass=[.01, .5] J/K  thermal_mass_Cauer=[.01, .1, .5] J/K  thermal_mass_Foster=[.001, .005, .05, .5] J/K  thermal_time_constant=[.001, .2] s  thermal_time_constant_Cauer=[.001, .1, .2] s  thermal_time_constant_Foster=[7e-05, .0007, .01, .08] s  thermal_mass_initial_temperatures=[25, 25] degC  thermal_mass_initial_temperatures_Cauer=[25, 25, 25] degC  junction_thermal_mass=0.01 J/K  Tvec_initial_Foster=[25, 25, 25, 25] degC  no_thermal_network=0  junction_temperature_specify=off  junction_temperature_priority=None  junction_temperature=25 degC  junction_temperature_nominal_specify=off  junction_temperature_nominal_value=1  junction_temperature_nominal_unit=degC  Qj_specify=off  Qj_priority=None  Qj=0 W  Qj_nominal_specify=off  Qj_nominal_value=1  Qj_nominal_unit=W  accumulatedSwitchingLosses_specify=off  accumulatedSwitchingLosses_priority=None  accumulatedSwitchingLosses=0 J
      settings: InternalSimscapePortConfiguration="{\"Bottom\":[],\"Left\":[{\"id\":\"G_elec\",\"label\":\"\",\"type\":\"foundation.electrical.electrical\"}],\"Right\":[{\"id\":\"C\",\"label\":\"\",\"type\":\"foundation.electrical.electrical\"},{\"id\":\"E\",\"label\":\"\",\"type\":\"foundation.electrical.electrical\"}],\"Top\":[]}"
  "IGBT (Ideal, Switching)1" : ee_lib/Semiconductors & Converters/IGBT (Ideal, Switching)  port_option=ee.enum.controlport.elec  Vf=0.8 V  Ron=0.001 Ohm  Goff=1e-5 1/Ohm  Vth=0.5 V  diode_param=ee.enum.semiconductors.protectionDiode.nodynamics  diode_Vf=0.8 V  diode_Ron=0.001 Ohm  diode_Goff=1e-5 1/Ohm  diode_C=50e-9 F  diode_iRM=-235 A  diode_iF=300 A  diode_idot=-50 A/us  diode_trr_param=ee.enum.converters.diodeReverseParam.trr_factor  diode_trr_factor=3  diode_trr=15 us  diode_Qrr=1500 s*uA  ice_specify=off  ice_priority=None  ice=0 A  ice_nominal_specify=off  ice_nominal_value=1  ice_nominal_unit=A  vce_specify=off  vce_priority=None  vce=0 V  vce_nominal_specify=off  vce_nominal_value=1  vce_nominal_unit=V  vge_specify=off  vge_priority=None  vge=0 V  vge_nominal_specify=off  vge_nominal_value=1  vge_nominal_unit=V  thermal_loss_option=ee.enum.converters.thermalLossOption.constantvalues  Von_data=[0, .1, .6, .8, 1, 1.3, 1.6, 2, 2.4; 0, .1, .7, 1, 1.2, 1.5, 1.9, 2.4, 2.8] V  Tj=[298.15, 398.15] K  Iout_data=[0, .1, 1, 5, 10, 20, 40, 70, 100] A  Eon_data=[0, .0024, .024, .12, .2, .48, 1.04, 2.16, 3.24; 0, .003, .03, .15, .25, .6, 1.3, 2.7, 4.05] * 1e-3 J  Eoff_data=[0, .0007, .0066, .033, .066, .17, .33, .83, 1.5; 0, .001, .01, .05, .1, .25, .5, 1.2, 2.2] * 1e-3 J  Eon_data_3D=[zeros(2, 9, 3)] J  Eoff_data_3D=[zeros(2, 9, 3)] J  Tj_loss=[298.15, 398.15] K  Iout_data_loss=[0, .1, 1, 5, 10, 20, 40, 70, 100] A  tabulateWithVce=false  Vce_loss=[0, 150, 300] V  Eon_scalar=22.86e-3 J  Eoff_scalar=17.14e-3 J  Voff=300 V  Iout_scalar=600 A  useCurrentFromPreviousCycle=false  useVoltageFromPreviousCycle=false  diodeModelType=ee.enum.converters.diodeModelType.pwl  diodeTableType=ee.enum.diode.tableType.IfMat  diode_ReverseIVType=ee.enum.diode.diodeReverseIV.constant  diode_IfMat=[.07, .12, .19, 1.75, 4.24, 7.32, 11.2; .16, .3, .72, 2.14, 4.02, 6.35, 9.12] A  diode_VfMat=[.9, 1.15, 1.25, 1.5, 1.75, 2.17, 2.6, 2.85; .58, .68, .75, 1.1, 1.38, 1.77, 2.27, 2.7] V  diode_TjVec=[25, 125] degC  diode_VfVec=[.5, .7, .9, 1.3, 1.7, 2.1, 2.5] V  diode_IfVec=[.1, .2, .5, 1, 2, 4, 7, 10] A  diode_IrMat=[1e-06, 2e-06, 5e-06, 1e-05, 2.5e-05, 5e-05, .0001; 2e-06, 5e-06, 1e-05, 4e-05, 8e-05, .0002, .0005] A  diode_VrMat=[10, 100, 200, 250, 300, 325, 350; 10, 70, 160, 220, 270, 300, 320] V  diode_VrVec=[10, 20, 40, 50, 70, 80, 100] V  diode_IrVec=[1e-06, 2e-06, 5e-06, 1e-05, 2e-05, 5e-05, .0001] A  diode_Vr=-600 V  diode_Ls=150 nH  diode_Erec=0.03 J  diode_rec_loss_model=ee.enum.diode.reverseRecoveryModel.fixed  diode_ErecVal=0 J  diode_scaleWithIandV=true  diode_ErecMat=zeros(2, 3) J  diode_TjrecVec=[298.15, 398.15] K  diode_IfrecVec=[.1, 1, 10] A  diode_IrecVal=10 A  diode_VrecVal=10 V  diode_tFilter=1 / 1000 / 100 s  thermal_network_parameterization=ee.enum.thermalNetworkTopology.external  Rth=[.08, .5] K/W  Rth_Cauer=[.08, .1, .5] K/W  Rth_Foster=[.08, .14, .22, .16] K/W  thermal_mass_parameterization=ee.enum.thermalNetwork.timeconstant  thermal_mass=[.01, .5] J/K  thermal_mass_Cauer=[.01, .1, .5] J/K  thermal_mass_Foster=[.001, .005, .05, .5] J/K  thermal_time_constant=[.001, .2] s  thermal_time_constant_Cauer=[.001, .1, .2] s  thermal_time_constant_Foster=[7e-05, .0007, .01, .08] s  thermal_mass_initial_temperatures=[25, 25] degC  thermal_mass_initial_temperatures_Cauer=[25, 25, 25] degC  junction_thermal_mass=0.01 J/K  Tvec_initial_Foster=[25, 25, 25, 25] degC  no_thermal_network=0  junction_temperature_specify=off  junction_temperature_priority=None  junction_temperature=25 degC  junction_temperature_nominal_specify=off  junction_temperature_nominal_value=1  junction_temperature_nominal_unit=degC  Qj_specify=off  Qj_priority=None  Qj=0 W  Qj_nominal_specify=off  Qj_nominal_value=1  Qj_nominal_unit=W  accumulatedSwitchingLosses_specify=off  accumulatedSwitchingLosses_priority=None  accumulatedSwitchingLosses=0 J
      settings: InternalSimscapePortConfiguration="{\"Bottom\":[],\"Left\":[{\"id\":\"G_elec\",\"label\":\"\",\"type\":\"foundation.electrical.electrical\"}],\"Right\":[{\"id\":\"C\",\"label\":\"\",\"type\":\"foundation.electrical.electrical\"},{\"id\":\"E\",\"label\":\"\",\"type\":\"foundation.electrical.electrical\"}],\"Top\":[]}"
  PS-Simulink Converter1 : nesl_utility/PS-Simulink Converter  PhysicalDomain=network_engine_domain  SubClassName=ps_output  LeftPortType=input  RightPortType=output  PseudoPeriodic=off  Frequencies=[]  VectorFormat=inherit  Unit=inherit  AffineConversion=off
  PS-Simulink Converter2 : nesl_utility/PS-Simulink Converter  PhysicalDomain=network_engine_domain  SubClassName=ps_output  LeftPortType=input  RightPortType=output  PseudoPeriodic=off  Frequencies=[]  VectorFormat=inherit  Unit=inherit  AffineConversion=off
  Scope1 : Scope
  Scope2 : Scope
  Voltage Sensor : fl_lib/Electrical/Electrical Sensors/Voltage Sensor
  Voltage Sensor1 : fl_lib/Electrical/Electrical Sensors/Voltage Sensor
  + : PMIOPort  Side=Left
  Phase : PMIOPort  Port=2  Side=Right
  HO : PMIOPort  Port=3  Side=Left
  LO : PMIOPort  Port=4  Side=Left
  - : PMIOPort  Port=5  Side=Left
  wires:
  PS-Simulink Converter2/1 -> Scope2/1
  PS-Simulink Converter1/1 -> Scope1/1
  connections:
  "IGBT (Ideal, Switching)1"/LConn1 -- LO/RConn1
  "IGBT (Ideal, Switching)"/RConn1 -- Voltage Sensor/LConn1 -- +/RConn1
  "IGBT (Ideal, Switching)"/LConn1 -- HO/RConn1
  -/RConn1 -- "IGBT (Ideal, Switching)1"/RConn2
  "IGBT (Ideal, Switching)"/RConn2 -- Voltage Sensor1/LConn1 -- "IGBT (Ideal, Switching)1"/RConn1 -- Phase/RConn1
  Voltage Sensor/RConn2 -- Electrical Reference3/LConn1
  Voltage Sensor/RConn1 -- PS-Simulink Converter2/LConn1
  Voltage Sensor1/RConn2 -- Electrical Reference1/LConn1
  Voltage Sensor1/RConn1 -- PS-Simulink Converter1/LConn1

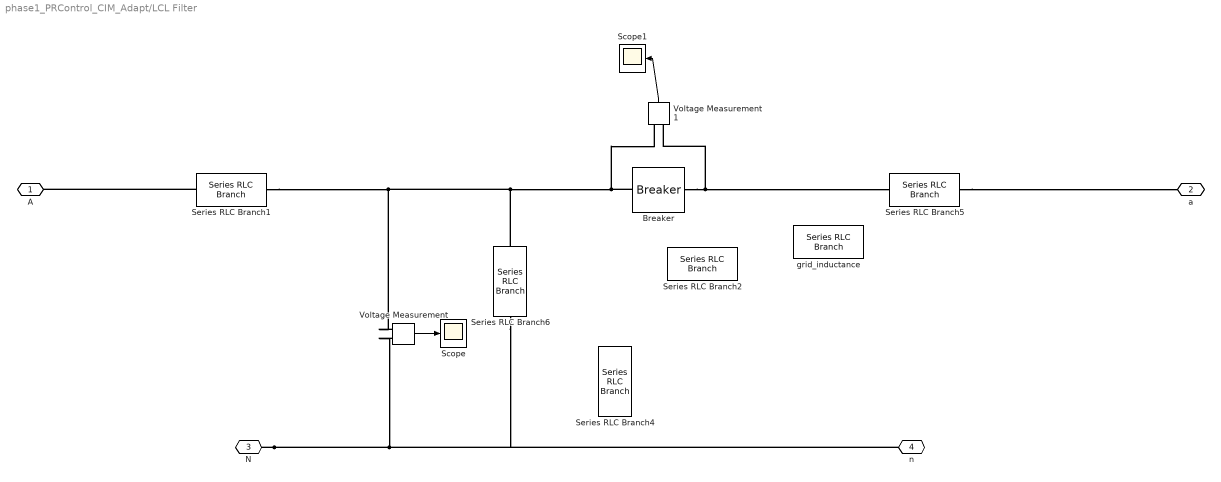
== system phase1_PRControl_CIM_Adapt/LCL Filter ==
  Breaker : spsBreakerLib/Breaker  InitialState=0  SwitchingTimes=[0]  External=off  BreakerResistance=0.0001  SnubberResistance=1e8  SnubberCapacitance=inf  Measurements=None  MoreParameters=on  NoBreakLoop=off
  Scope : Scope
  Scope1 : Scope
  Series RLC Branch1 : spsSeriesRLCBranchLib/Series RLC Branch  LConnTagsString=__new0  RConnTagsString=__new0  BranchType=RL  Resistance=R1  Inductance=L1  SetiL0=off  InitialCurrent=0  Capacitance=1e-6  Setx0=off  InitialVoltage=0  Measurements=None
  Series RLC Branch2 : spsSeriesRLCBranchLib/Series RLC Branch  LConnTagsString=__new0  RConnTagsString=__new0  BranchType=R  Resistance=0.135  Inductance=500e-6  SetiL0=off  InitialCurrent=0  Capacitance=1e-6  Setx0=off  InitialVoltage=0  Measurements=None
  Series RLC Branch4 : spsSeriesRLCBranchLib/Series RLC Branch  LConnTagsString=__new0  RConnTagsString=__new0  BranchType=R  Resistance=1  Inductance=500e-6  SetiL0=off  InitialCurrent=0  Capacitance=1e-6  Setx0=off  InitialVoltage=0  Measurements=None
  Series RLC Branch5 : spsSeriesRLCBranchLib/Series RLC Branch  LConnTagsString=__new0  RConnTagsString=__new0  BranchType=RL  Resistance=R2g  Inductance=L2g  SetiL0=off  InitialCurrent=0  Capacitance=1e-6  Setx0=off  InitialVoltage=0  Measurements=None
  Series RLC Branch6 : spsSeriesRLCBranchLib/Series RLC Branch  LConnTagsString=__new0  RConnTagsString=__new0  BranchType=RC  Resistance=Rd  Inductance=500e-6  SetiL0=off  InitialCurrent=0  Capacitance=Cf  Setx0=off  InitialVoltage=0  Measurements=None
  Voltage Measurement : spsVoltageMeasurementLib/Voltage Measurement  PhasorSimulation=off  OutputType=Complex  PSBequivalent=0
  Voltage Measurement1 : spsVoltageMeasurementLib/Voltage Measurement  PhasorSimulation=off  OutputType=Complex  PSBequivalent=0
  grid_inductance : spsSeriesRLCBranchLib/Series RLC Branch  LConnTagsString=__new0  RConnTagsString=__new0  BranchType=RL  Resistance=0  Inductance=5e-3  SetiL0=off  InitialCurrent=0  Capacitance=1e-6  Setx0=off  InitialVoltage=0  Measurements=None
  A : PMIOPort  Side=Left
  a : PMIOPort  Port=2  Side=Right
  N : PMIOPort  Port=3  Side=Left
  n : PMIOPort  Port=4  Side=Right
  wires:
  Voltage Measurement1/1 -> Scope1/1
  Voltage Measurement/1 -> Scope/1
  connections:
  N/RConn1 -- Series RLC Branch6/LConn1 -- n/RConn1 -- Voltage Measurement/LConn2
  Series RLC Branch5/RConn1 -- a/RConn1
  Series RLC Branch1/LConn1 -- A/RConn1
  Series RLC Branch6/RConn1 -- Voltage Measurement1/LConn2 -- Breaker/LConn1 -- Voltage Measurement/LConn1 -- Series RLC Branch1/RConn1
  Breaker/RConn1 -- Series RLC Branch5/LConn1 -- Voltage Measurement1/LConn1

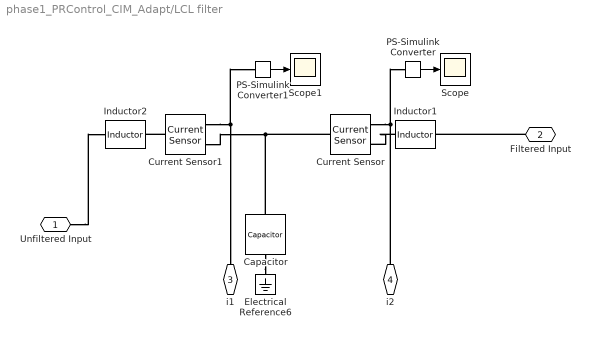
== system phase1_PRControl_CIM_Adapt/LCL filter ==
  Capacitor : fl_lib/Electrical/Electrical Elements/Capacitor  c=C_filter F  r=1e-6 Ohm  g=0 1/Ohm  i_specify=off  i_priority=None  i=0 A  i_nominal_specify=off  i_nominal_value=1  i_nominal_unit=A  v_specify=off  v_priority=None  v=0 V  v_nominal_specify=off  v_nominal_value=1  v_nominal_unit=V  vc_specify=off  vc_priority=High  vc=0 V  vc_nominal_specify=off  vc_nominal_value=1  vc_nominal_unit=V
  Current Sensor : fl_lib/Electrical/Electrical Sensors/Current Sensor
  Current Sensor1 : fl_lib/Electrical/Electrical Sensors/Current Sensor
  Electrical Reference6 : fl_lib/Electrical/Electrical Elements/Electrical Reference
  Inductor1 : fl_lib/Electrical/Electrical Elements/Inductor  l=1.5e-3 H  r=0 Ohm  g=1e-9 1/Ohm  i_specify=off  i_priority=None  i=0 A  i_nominal_specify=off  i_nominal_value=1  i_nominal_unit=A  v_specify=off  v_priority=None  v=0 V  v_nominal_specify=off  v_nominal_value=1  v_nominal_unit=V  i_L_specify=off  i_L_priority=High  i_L=0 A  i_L_nominal_specify=off  i_L_nominal_value=1  i_L_nominal_unit=A
  Inductor2 : fl_lib/Electrical/Electrical Elements/Inductor  l=1.5e-3 H  r=0 Ohm  g=1e-9 1/Ohm  i_specify=off  i_priority=None  i=0 A  i_nominal_specify=off  i_nominal_value=1  i_nominal_unit=A  v_specify=off  v_priority=None  v=0 V  v_nominal_specify=off  v_nominal_value=1  v_nominal_unit=V  i_L_specify=off  i_L_priority=High  i_L=0 A  i_L_nominal_specify=off  i_L_nominal_value=1  i_L_nominal_unit=A
  PS-Simulink Converter : nesl_utility/PS-Simulink Converter  PhysicalDomain=network_engine_domain  SubClassName=ps_output  LeftPortType=input  RightPortType=output  PseudoPeriodic=off  Frequencies=[]  VectorFormat=inherit  Unit=inherit  AffineConversion=off
  PS-Simulink Converter1 : nesl_utility/PS-Simulink Converter  PhysicalDomain=network_engine_domain  SubClassName=ps_output  LeftPortType=input  RightPortType=output  PseudoPeriodic=off  Frequencies=[]  VectorFormat=inherit  Unit=inherit  AffineConversion=off
  Scope : Scope
  Scope1 : Scope
  Unfiltered Input : PMIOPort  Side=Left
  Filtered Input : PMIOPort  Port=2  Side=Right
  i1 : PMIOPort  Port=3  Side=Right
  i2 : PMIOPort  Port=4  Side=Right
  wires:
  PS-Simulink Converter/1 -> Scope/1
  PS-Simulink Converter1/1 -> Scope1/1
  connections:
  Inductor1/RConn1 -- Current Sensor/RConn2
  Current Sensor/RConn1 -- PS-Simulink Converter/LConn1 -- i2/RConn1
  Filtered Input/RConn1 -- Inductor1/LConn1
  Capacitor/LConn1 -- Current Sensor/LConn1 -- Current Sensor1/RConn2
  Unfiltered Input/RConn1 -- Inductor2/RConn1
  Current Sensor1/RConn1 -- i1/RConn1 -- PS-Simulink Converter1/LConn1
  Capacitor/RConn1 -- Electrical Reference6/LConn1
  Current Sensor1/LConn1 -- Inductor2/LConn1

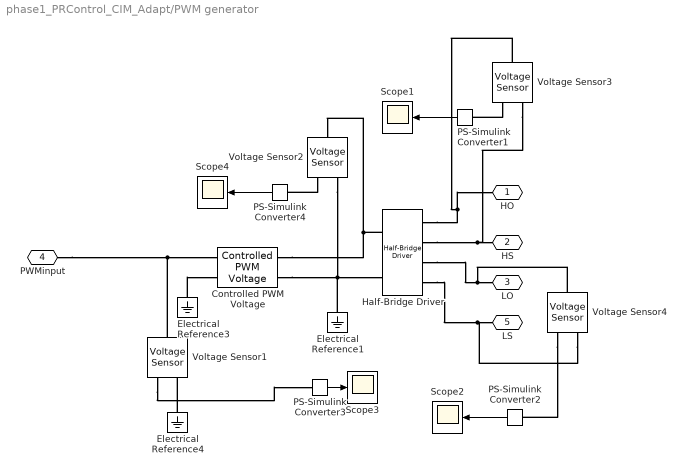
== system phase1_PRControl_CIM_Adapt/PWM generator ==
  Controlled PWM Voltage : ee_lib/Integrated Circuits/Controlled PWM Voltage  F=16000 Hz  TD=0 s  pulse_width_offset=0 s  pulse_min=0 s  pwm_or_av=ee.enum.pwm_or_av.pwm  event_type=ee.enum.ic.event.asynchronous  sample_time=1e-6 s  Vmin=0 V  Vmax=1 V  Vm=1 V  u_min=0  u_max=1
  Electrical Reference1 : fl_lib/Electrical/Electrical Elements/Electrical Reference
  Electrical Reference3 : fl_lib/Electrical/Electrical Elements/Electrical Reference
  Electrical Reference4 : fl_lib/Electrical/Electrical Elements/Electrical Reference
  Half-Bridge Driver : ee_lib/Semiconductors & Converters/Half-Bridge Driver  port_option=ee.enum.controlport.elec  uHigh=0.55 V  uLow=0.45 V  uHighValue=0.7  uLowValue=0.3  vHigh=1 V  vLow=0 V  tpLH=50 ns  tdLH=100 ns  tpHL=50 ns  tdHL=100 ns  parameterization=ee.enum.semiconductors.gateDriverParam.riseAndFallTimes  rHigh=2 Ohm  rLow=2 Ohm  tRise=20 ns  tFall=20 ns  cLoad=10 nF  enable_faults=simscape.enum.onoff.off  t_fault=1 s  fault_type=ee.enum.semiconductors.halfBridgeDriverFault.failInput0  ZonTime_specify=off  ZonTime_priority=None  ZonTime=0 s  ZoffTime_specify=off  ZoffTime_priority=None  ZoffTime=0 s  power_dissipated_high_side_specify=off  power_dissipated_high_side_priority=None  power_dissipated_high_side=0 W  power_dissipated_high_side_nominal_specify=off  power_dissipated_high_side_nominal_value=1  power_dissipated_high_side_nominal_unit=W  power_dissipated_low_side_specify=off  power_dissipated_low_side_priority=None  power_dissipated_low_side=0 W  power_dissipated_low_side_nominal_specify=off  power_dissipated_low_side_nominal_value=1  power_dissipated_low_side_nominal_unit=W
      settings: InternalSimscapePortConfiguration="{\"Bottom\":[],\"Left\":[{\"id\":\"PWM\",\"label\":\"PWM\",\"type\":\"foundation.electrical.electrical\"},{\"id\":\"REF\",\"label\":\"REF\",\"type\":\"foundation.electrical.electrical\"}],\"Right\":[{\"id\":\"HO\",\"label\":\"HO\",\"type\":\"foundation.electrical.electrical\"},{\"id\":\"HS\",\"label\":\"HS\",\"type\":\"foundation.electrical.electrical\"},{\"id\":\"LO\",\"label\":\"LO\",\"type\":\"foundation.electrical.electrical\"},{\"id\":\"LS\",\"label\":\"LS\",\"type\":\"foundation.electrical.electrical\"}],\"Top\":[]}"
  PS-Simulink Converter{1..4} (4 alike) : nesl_utility/PS-Simulink Converter  PhysicalDomain=network_engine_domain  SubClassName=ps_output  LeftPortType=input  RightPortType=output  PseudoPeriodic=off  Frequencies=[]  VectorFormat=inherit  Unit=inherit  AffineConversion=off
  Scope{1..4} (4 alike) : Scope
  Voltage Sensor{1..4} (4 alike) : fl_lib/Electrical/Electrical Sensors/Voltage Sensor
  HO : PMIOPort  Side=Right
  HS : PMIOPort  Port=2  Side=Right
  LO : PMIOPort  Port=3  Side=Right
  PWMinput : PMIOPort  Port=4  Side=Left
  LS : PMIOPort  Port=5  Side=Right
  wires:
  PS-Simulink Converter4/1 -> Scope4/1
  PS-Simulink Converter3/1 -> Scope3/1
  PS-Simulink Converter1/1 -> Scope1/1
  PS-Simulink Converter2/1 -> Scope2/1
  connections:
  Electrical Reference3/LConn1 -- Controlled PWM Voltage/LConn2
  Electrical Reference4/LConn1 -- Voltage Sensor1/RConn2
  Half-Bridge Driver/RConn4 -- Voltage Sensor4/RConn2 -- LS/RConn1
  Controlled PWM Voltage/RConn2 -- Electrical Reference1/LConn1 -- Voltage Sensor2/RConn2 -- Half-Bridge Driver/LConn2
  Voltage Sensor1/LConn1 -- PWMinput/RConn1 -- Controlled PWM Voltage/LConn1
  Voltage Sensor2/RConn1 -- PS-Simulink Converter4/LConn1
  Half-Bridge Driver/RConn2 -- Voltage Sensor3/RConn2 -- HS/RConn1
  Controlled PWM Voltage/RConn1 -- Voltage Sensor2/LConn1 -- Half-Bridge Driver/LConn1
  Half-Bridge Driver/RConn3 -- Voltage Sensor4/LConn1 -- LO/RConn1
  Half-Bridge Driver/RConn1 -- Voltage Sensor3/LConn1 -- HO/RConn1
  Voltage Sensor1/RConn1 -- PS-Simulink Converter3/LConn1
  Voltage Sensor3/RConn1 -- PS-Simulink Converter1/LConn1
  Voltage Sensor4/RConn1 -- PS-Simulink Converter2/LConn1

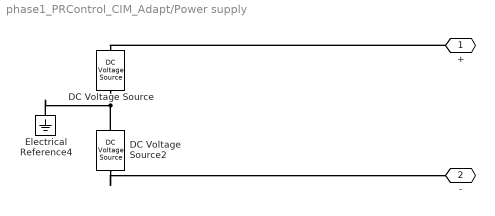
== system phase1_PRControl_CIM_Adapt/Power supply ==
  DC Voltage Source : ee_lib/Additional Components/SPICE Sources/DC Voltage Source  DC=370 V
  DC Voltage Source2 : ee_lib/Additional Components/SPICE Sources/DC Voltage Source  DC=370 V
  Electrical Reference4 : fl_lib/Electrical/Electrical Elements/Electrical Reference
  + : PMIOPort  Side=Right
  - : PMIOPort  Port=2  Side=Right
  connections:
  DC Voltage Source2/RConn1 -- -/RConn1
  +/RConn1 -- DC Voltage Source/LConn1
  Electrical Reference4/LConn1 -- DC Voltage Source/RConn1 -- DC Voltage Source2/LConn1
